simulink model "simulink_model"  (R2013a)
settings: Solver=VariableStepDiscrete  StartTime=0.0  StopTime=inf  RelTol=1e-3
undefined symbols (not defined in the file): fdesignblkfcn, gcbh
libraries: dspsigops x4, simulink x3
settings Model: Creator=franz  LastModifiedBy=franz

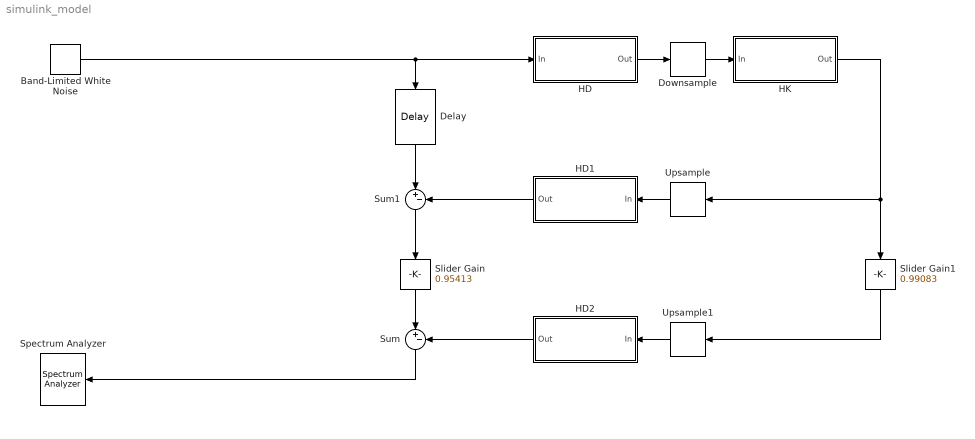
== system simulink_model ==
  Band-Limited White Noise : simulink/Sources/Band-Limited White Noise  Cov=[0.5]  Ts=1/44e3  seed=[23341]
  Delay : dspsigops/Delay  InputProcessing=Columns as channels (frame based)  dly_unit=Samples  delay=13+13+2*29  ic_detail=off  dif_ic_for_ch=off  dif_ic_for_dly=off  ic=0  reset_popup=None
  Downsample : dspsigops/Downsample  N=2  phase=0  RateOptions=Allow multirate processing  smode=Allow multirate  fmode=Maintain input frame size  ic=0
  HD : Subsystem  DialogController=fdesignblkfcn  InitFcn=fdesignblkfcn(gcbh, {'InitFcn'});  mask(Lowpass Filter){}
      mask help: Design a lowpass filter
      settings: CopyFcn=fdesignblkfcn(gcbh, {'CopyFcn'});
      mask Help: helpview(mapfilelocation('dsp'), 'dsplowpassfilter');
      mask Display: disp('Lowpass')
  HD1 : Subsystem  DialogController=fdesignblkfcn  InitFcn=fdesignblkfcn(gcbh, {'InitFcn'});  mask(Lowpass Filter){}
      mask help: Design a lowpass filter
      settings: CopyFcn=fdesignblkfcn(gcbh, {'CopyFcn'});
      mask Help: helpview(mapfilelocation('dsp'), 'dsplowpassfilter');
      mask Display: disp('Lowpass')
  HD2 : Subsystem  DialogController=fdesignblkfcn  InitFcn=fdesignblkfcn(gcbh, {'InitFcn'});  mask(Lowpass Filter){}
      mask help: Design a lowpass filter
      settings: CopyFcn=fdesignblkfcn(gcbh, {'CopyFcn'});
      mask Help: helpview(mapfilelocation('dsp'), 'dsplowpassfilter');
      mask Display: disp('Lowpass')
  HK : Subsystem  DialogController=fdesignblkfcn  InitFcn=fdesignblkfcn(gcbh, {'InitFcn'});  mask(Lowpass Filter){}
      mask help: Design a lowpass filter
      settings: CopyFcn=fdesignblkfcn(gcbh, {'CopyFcn'});
      mask Help: helpview(mapfilelocation('dsp'), 'dsplowpassfilter');
      mask Display: disp('Lowpass')
  Slider Gain : simulink/Math Operations/Slider Gain  low=0  gain=0.95413  high=2
  Slider Gain1 : simulink/Math Operations/Slider Gain  low=0  gain=0.99083  high=2
  Spectrum Analyzer : SpectrumAnalyzer
      settings: CopyFcn=scopeextensions.ScopeBlock.callback(gcbh, 'onBlockCopy', gcbh);  DeleteFcn=scopeextensions.ScopeBlock.callback(gcbh, 'onBlockDelete');  PreSaveFcn=scopeextensions.ScopeBlock.callback(gcbh, 'onModelSave');  NameChangeFcn=scopeextensions.ScopeBlock.callback(gcbh, 'onBlockRename');  CloseFcn=scopeextensions.ScopeBlock.callback(gcbh, 'onBlockClose');  PreDeleteFcn=scopeextensions.ScopeBlock.callback(gcbh, 'onBlockPreDelete');
  Sum : Sum  Inputs=|+-
  Sum1 : Sum  Inputs=|+-
  Upsample : dspsigops/Upsample  N=2  phase=0  RateOptions=Allow multirate processing  ic=0  mode=Unused parameter value
  Upsample1 : dspsigops/Upsample  N=2  phase=0  RateOptions=Allow multirate processing  ic=0  mode=Unused parameter value
  wires:
  HD/1(Out) -> Downsample/1
  Downsample/1 -> HK/1(In)
  Band-Limited White Noise/1 -> Delay/1, HD/1(In)
  Upsample/1 -> HD1/1(In)
  Upsample1/1 -> HD2/1(In)
  HK/1(Out) -> Slider Gain1/1, Upsample/1
  Delay/1 -> Sum1/1
  HD1/1(Out) -> Sum1/2
  Sum1/1 -> Slider Gain/1
  HD2/1(Out) -> Sum/2
  Sum/1 -> Spectrum Analyzer/1
  Slider Gain/1 -> Sum/1
  Slider Gain1/1 -> Upsample1/1

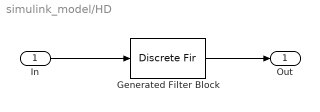
== system simulink_model/HD ==
  In : Inport
  Generated Filter Block : DiscreteFir  Tag=BlockMethodSubSystem  FilterStructure=Direct form symmetric  Coefficients=[0.00125499973307861574 7.5121006642194005e-06 -0.00440618438867188683 0.000306790345692007119 0.0107352745210879605 -0.000531534917778082113 -0.0229010335041911935 0.00101598787352332582 0.0452490731992706424 -0.00135780658931751301 -0.0940901325308465403 0.00171431710826016638 0.314088582190462762 0.498226932007327927 0.314088582190462762 0.00171431710826016638 -0.0940901325308465403 -0.00135780658931751301 0.0452490731992706424 0.00101598787352332582 -0.0229010335041911935 -0.000531534917778082113 0.0107352745210879605 0.000306790345692007119 -0.00440618438867188683 7.5121006642194005e-06 0.00125499973307861574]  InputProcessing=Columns as channels (frame based)
  Out : Outport
  wires:
  In/1 -> Generated Filter Block/1
  Generated Filter Block/1 -> Out/1

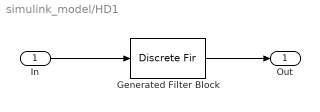
== system simulink_model/HD1 ==
  In : Inport
  Generated Filter Block : DiscreteFir  Tag=BlockMethodSubSystem  FilterStructure=Direct form symmetric  Coefficients=[0.00125499973307861574 7.5121006642194005e-06 -0.00440618438867188683 0.000306790345692007119 0.0107352745210879605 -0.000531534917778082113 -0.0229010335041911935 0.00101598787352332582 0.0452490731992706424 -0.00135780658931751301 -0.0940901325308465403 0.00171431710826016638 0.314088582190462762 0.498226932007327927 0.314088582190462762 0.00171431710826016638 -0.0940901325308465403 -0.00135780658931751301 0.0452490731992706424 0.00101598787352332582 -0.0229010335041911935 -0.000531534917778082113 0.0107352745210879605 0.000306790345692007119 -0.00440618438867188683 7.5121006642194005e-06 0.00125499973307861574]  InputProcessing=Columns as channels (frame based)
  Out : Outport
  wires:
  In/1 -> Generated Filter Block/1
  Generated Filter Block/1 -> Out/1

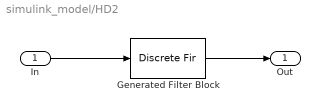
== system simulink_model/HD2 ==
  In : Inport
  Generated Filter Block : DiscreteFir  Tag=BlockMethodSubSystem  FilterStructure=Direct form symmetric  Coefficients=[0.00125499973307861574 7.5121006642194005e-06 -0.00440618438867188683 0.000306790345692007119 0.0107352745210879605 -0.000531534917778082113 -0.0229010335041911935 0.00101598787352332582 0.0452490731992706424 -0.00135780658931751301 -0.0940901325308465403 0.00171431710826016638 0.314088582190462762 0.498226932007327927 0.314088582190462762 0.00171431710826016638 -0.0940901325308465403 -0.00135780658931751301 0.0452490731992706424 0.00101598787352332582 -0.0229010335041911935 -0.000531534917778082113 0.0107352745210879605 0.000306790345692007119 -0.00440618438867188683 7.5121006642194005e-06 0.00125499973307861574]  InputProcessing=Columns as channels (frame based)
  Out : Outport
  wires:
  In/1 -> Generated Filter Block/1
  Generated Filter Block/1 -> Out/1

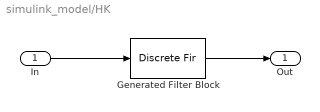
== system simulink_model/HK ==
  In : Inport
  Generated Filter Block : DiscreteFir  Tag=BlockMethodSubSystem  Coefficients=[-0.000304826338356967727 0.000846681314782982944 -0.000265927185337464834 -0.000778113926763290657 0.00160273093866428987 -0.00066269986872389804 -0.00170938786067070152 0.00312395681211410231 -0.00116234706548520427 -0.00324555673293471262 0.00551263910028795389 -0.00178513128518868356 -0.00572135794270587153 0.00908358083374183854 -0.00249420413816246441 -0.00962676825397603894 0.0143671301277249648 -0.00322923830265499281 -0.0158687064538101351 0.0224640231986175977 -0.00391559299688197873 -0.0265938643613188135 0.0363637715113083737 -0.00447623295304109062 -0.0490200264581345177 0.0682146163606980049 -0.00484305817633839692 -0.133815711588658154 0.27736017788785633 0.661695990092098341 0.27736017788785633 -0.133815711588658154 -0.00484305817633839692 0.0682146163606980049 -0.0490200264581345177 -0.00447623295304109062 0.0363637715113083737 -0.0265938643613188135 -0.00391559299688197873 0.0224640231986175977 -0.0158687064538101351 -0.00322923830265499281 0.0143671301277249648 -0.00962676825397603894 -0.00249420413816246441 0.00908358083374183854 -0.00572135794270587153 -0.00178513128518868356 0.00551263910028795389 -0.00324555673293471262 -0.00116234706548520427 0.00312395681211410231 -0.00170938786067070152 -0.00066269986872389804 0.00160273093866428987 -0.000778113926763290657 -0.000265927185337464834 0.000846681314782982944 -0.000304826338356967727]  InputProcessing=Columns as channels (frame based)
  Out : Outport
  wires:
  In/1 -> Generated Filter Block/1
  Generated Filter Block/1 -> Out/1
